simulink model "pacemaker"  (R2020a)
settings: Solver=FixedStepAuto  StartTime=0.0  StopTime=10.0  FixedStep=1e-3  RelTol=1e-3  EnableMultiTasking=on
undefined symbols (not defined in the file): A0, A1, D0, D1, D10, D11, D12, D13, D2, D3, D4, D5, D6, D7, D8, D9, PTA0, PTA1, PTA2, PTB2, PTB23, PTB3, PTB9, PTC16, PTC17, PTC2, PTC3, PTC4, PTD0, PTD1, PTD2, PTD3
libraries: frdmk64flib x22, etargetslib x8
settings Model: ExtModeTrigDuration=5  Creator=V  LastModifiedBy=V
settings OptimizationCC: EnhancedBackFolding=on  PassReuseOutputArgsAs=Individual arguments  ZeroExternalMemoryAtStartup=off  ZeroInternalMemoryAtStartup=off  MaxStackSize=64  OptimizeBlockOrder=speed  DifferentSizesBufferReuse=on  OptimizationCustomize=off  EfficientTunableParamExpr=on
settings DebuggingCC: ParameterTunabilityLossMsg=error
settings HardwareCC: ProdBitPerPointer=32  ProdBitPerSizeT=32  ProdBitPerPtrDiffT=32  ProdLargestAtomicInteger=Long  ProdLargestAtomicFloat=Double  ProdWordSize=32  ProdHWDeviceType=ARM Compatible->ARM Cortex
settings SFSimCC: MATLABDynamicMemAlloc=off
settings RTWCC: SystemTargetFile=ert.tlc  HardwareBoard=NXP FRDM-K64F  TemplateMakefile=ert_default_tmf  Toolchain=GNU Tools for ARM Embedded Processors
settings CodeAppCC: ForceParamTrailComments=on  IgnoreCustomStorageClasses=off  OperatorAnnotations=on  SimulinkDataObjDesc=on  SFDataObjDesc=on  InsertBlockDesc=on

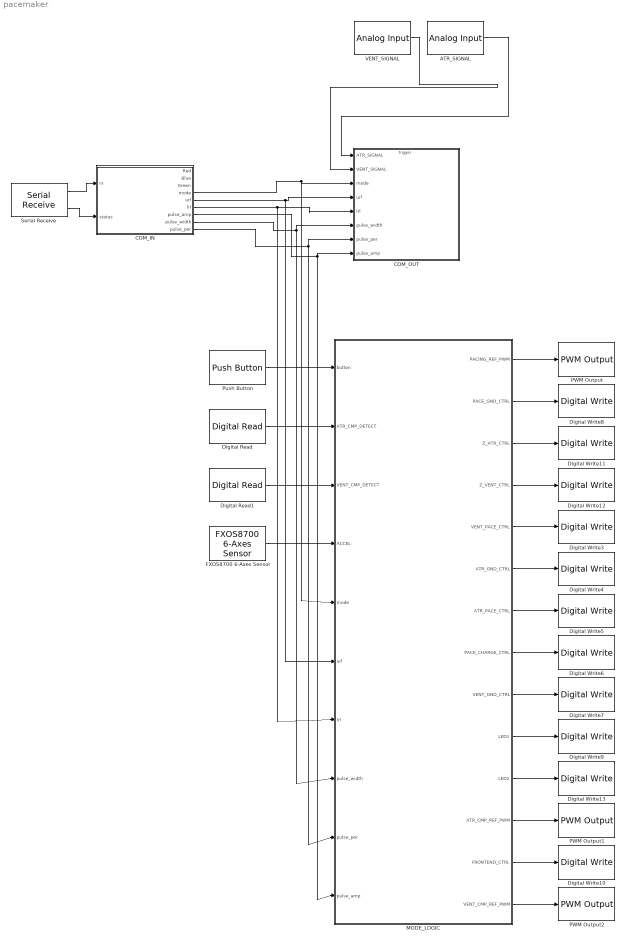
== system pacemaker ==
  ATR_SIGNAL : frdmk64flib/Analog Input  Whichpin=PTB2 (A0)  SampleTime=-1
  COM_IN : Stateflow chart  TreatAsAtomicUnit=on
      settings: PortSchema="{\"entries\":[{\"content\":{\"sides\":[{\"content\":{\"connectorIds\":[\"In2\",\"In1\"]},\"type\":\"ConnectorPlacement.EquallySpacedRectSide\",\"uuid\":\"8daf93b5-21b0-4142-b4ab-857b16f8f8fd\"},{\"content\":{\"connectorIds\":[\"Out1\",\"Out2\",\"Out3\",\"Out4\",\"Out5\",\"Out6\",\"Out7\",\"Out8\",\"Out9\"],\"side\":\"RIGHT\"},\"type\":\"ConnectorPlacement.EquallySpacedRectSide\",\"uuid\":\"6413e42a-ae9b-49fc-8e61-a3b5f4c35bed\"},{\"content\":{\"connectorIds\":[],\"side\":\"TOP\"},\"type\":\"ConnectorPlacement.EquallySpacedRectSide\",\"uuid\":\"39f92d96-10a7-4496-b9ea-08b56c7f9280\"}]},\"type\":\"ConnectorPlacement.EquallySpacedConnector\",\"uuid\":\"717f6531-5e3e-445a-90fb-8047e6ab3765\"}],\"packageUris\":[\"http://schema.mathworks.com/mf0/Connector/19700101\"],\"version\":\"1.0\"}"
  COM_OUT : Subsystem
  Digital Read : frdmk64flib/Digital Read  Whichpin=PTC16 (D0)  SampleTime=-1
  Digital Read1 : frdmk64flib/Digital Read  Whichpin=PTC17 (D1)  SampleTime=-1
  Digital Write10 : frdmk64flib/Digital Write  Whichpin=PTD1 (D13)
  Digital Write11 : frdmk64flib/Digital Write  Whichpin=PTB23 (D4)
  Digital Write12 : frdmk64flib/Digital Write  Whichpin=PTC3 (D7)
  Digital Write13 : frdmk64flib/Digital Write  Whichpin=GREEN_LED
  Digital Write3 : frdmk64flib/Digital Write  Whichpin=PTC4 (D9)
  Digital Write4 : frdmk64flib/Digital Write  Whichpin=PTD2 (D11)
  Digital Write5 : frdmk64flib/Digital Write  Whichpin=PTA0 (D8)
  Digital Write6 : frdmk64flib/Digital Write  Whichpin=PTB9 (D2)
  Digital Write7 : frdmk64flib/Digital Write  Whichpin=PTD3 (D12)
  Digital Write8 : frdmk64flib/Digital Write  Whichpin=PTD0 (D10)
  Digital Write9 : frdmk64flib/Digital Write  Whichpin=RED_LED
  FXOS8700 6-Axes Sensor : frdmk64flib/FXOS8700 6-Axes Sensor  Activesensor=Accelerometer only  ODR=800Hz  HybridODR=400Hz  Accelfullrange=-4g to +4g  SampleTime=-1
  MODE_LOGIC : Stateflow chart  TreatAsAtomicUnit=on
      settings: PortSchema="{\"entries\":[{\"content\":{\"sides\":[{\"content\":{\"connectorIds\":[\"In1\",\"In2\",\"In3\",\"In4\",\"In10\",\"In6\",\"In5\",\"In8\",\"In7\",\"In9\"]},\"type\":\"ConnectorPlacement.EquallySpacedRectSide\",\"uuid\":\"04414c83-1a99-45b4-b483-67b067b91455\"},{\"content\":{\"connectorIds\":[\"Out1\",\"Out2\",\"Out3\",\"Out4\",\"Out5\",\"Out6\",\"Out7\",\"Out8\",\"Out9\",\"Out10\",\"Out11\",\"Out12\",\"Out13\",\"Out14\"],\"side\":\"RIGHT\"},\"type\":\"ConnectorPlacement.EquallySpacedRectSide\",\"uuid\":\"10735fb8-9010-49d7-9ae9-fd379b89587a\"},{\"content\":{\"connectorIds\":[],\"side\":\"TOP\"},\"type\":\"ConnectorPlacement.EquallySpacedRectSide\",\"uuid\":\"3c1ca38a-0b4c-49c9-8ccc-830417faf6d4\"}]},\"type\":\"ConnectorPlacement.EquallySpacedConnector\",\"uuid\":\"9d19b875-14af-4a64-aa13-2b0c973f73dc\"}],\"packageUris\":[\"http://schema.mathworks.com/mf0/Connector/19700101\"],\"version\":\"1.0\"}"
  PWM Output : frdmk64flib/PWM Output  Whichpin=PTA2 (D5)  InitialFrequency=2000  InitialDutyCycle=70
  PWM Output1 : frdmk64flib/PWM Output  Whichpin=PTC2 (D6)  InitialFrequency=2000  InitialDutyCycle=50
  PWM Output2 : frdmk64flib/PWM Output  Whichpin=PTA1 (D3)  InitialFrequency=2000  InitialDutyCycle=50
  Push Button : frdmk64flib/Push Button  Whichswitch=SW2  SampleTime1=-1
  Serial Receive : frdmk64flib/Serial Receive  SCIModule=0  Baudrate=uint32(9600)  Parity=None  StopBits=1  HardwareFlowControl=None  ByteOrder=LittleEndian  DataType=uint8  DataLength=44  BlockingMode=off  OutputStatus=on  SampleTime=0.1
  VENT_SIGNAL : frdmk64flib/Analog Input  Whichpin=PTB3 (A1)  SampleTime=-1
  wires:
  Serial Receive/2 -> COM_IN/1(status)
  Serial Receive/1 -> COM_IN/2(rx)
  VENT_SIGNAL/1 -> COM_OUT/2(VENT_SIGNAL)
  ATR_SIGNAL/1 -> COM_OUT/1(ATR_SIGNAL)
  COM_IN/4(mode) -> MODE_LOGIC/10(mode), COM_OUT/3(mode)
  COM_IN/5(url) -> MODE_LOGIC/6(url), COM_OUT/4(url)
  COM_IN/6(lrl) -> MODE_LOGIC/5(lrl), COM_OUT/5(lrl)
  COM_IN/8(pulse_width) -> MODE_LOGIC/8(pulse_width), COM_OUT/6(pulse_width)
  COM_IN/7(pulse_amp) -> MODE_LOGIC/9(pulse_amp), COM_OUT/8(pulse_amp)
  COM_IN/9(pulse_per) -> MODE_LOGIC/7(pulse_per), COM_OUT/7(pulse_per)
  MODE_LOGIC/8(PACE_CHARGE_CTRL) -> Digital Write6/1
  MODE_LOGIC/10(LED1) -> Digital Write9/1
  MODE_LOGIC/6(ATR_GND_CTRL) -> Digital Write4/1
  MODE_LOGIC/13(FRONTEND_CTRL) -> Digital Write10/1
  MODE_LOGIC/2(PACE_GND_CTRL) -> Digital Write8/1
  MODE_LOGIC/9(VENT_GND_CTRL) -> Digital Write7/1
  MODE_LOGIC/14(VENT_CMP_REF_PWM) -> PWM Output2/1
  MODE_LOGIC/7(ATR_PACE_CTRL) -> Digital Write5/1
  MODE_LOGIC/1(PACING_REF_PWM) -> PWM Output/1
  MODE_LOGIC/11(LED2) -> Digital Write13/1
  MODE_LOGIC/12(ATR_CMP_REF_PWM) -> PWM Output1/1
  MODE_LOGIC/3(Z_ATR_CTRL) -> Digital Write11/1
  MODE_LOGIC/4(Z_VENT_CTRL) -> Digital Write12/1
  MODE_LOGIC/5(VENT_PACE_CTRL) -> Digital Write3/1
  Push Button/1 -> MODE_LOGIC/1(button)
  Digital Read/1 -> MODE_LOGIC/2(ATR_CMP_DETECT)
  Digital Read1/1 -> MODE_LOGIC/3(VENT_CMP_DETECT)
  FXOS8700 6-Axes Sensor/1 -> MODE_LOGIC/4(ACCEL)

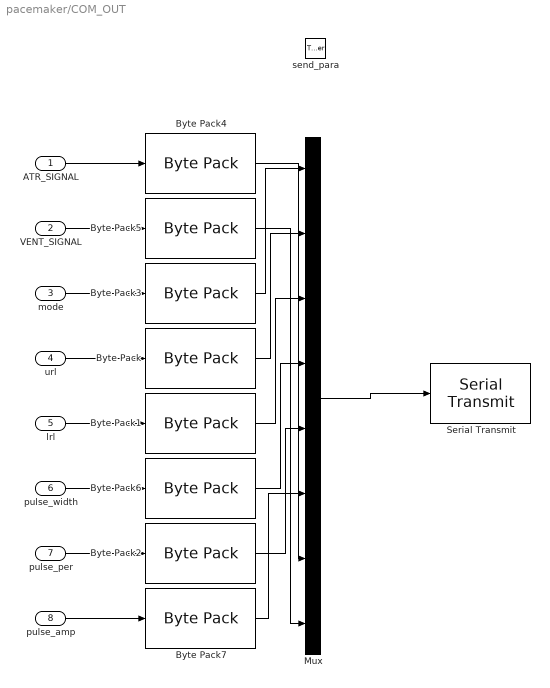
== system pacemaker/COM_OUT ==
  ATR_SIGNAL : Inport  OutDataTypeStr=double
  VENT_SIGNAL : Inport  Port=2  OutDataTypeStr=double
  mode : Inport  Port=3  OutDataTypeStr=uint16
  url : Inport  Port=4  OutDataTypeStr=double
  lrl : Inport  Port=5  OutDataTypeStr=double
  pulse_width : Inport  Port=6  OutDataTypeStr=double
  pulse_per : Inport  Port=7  OutDataTypeStr=double
  pulse_amp : Inport  Port=8  OutDataTypeStr=double
  send_para : TriggerPort  TriggerType=function-call  IsSimulinkFunction=on  FunctionName=send_para  VariantControl=Variant
  Byte Pack{,1..2,4..7} (7 alike) : etargetslib/Byte Pack  datatypes={'double'}  byteAlign=1
  Byte Pack3 : etargetslib/Byte Pack  datatypes={'uint16'}  byteAlign=1
  Mux : Mux  Inputs=8
  Serial Transmit : frdmk64flib/Serial Transmit  SCIModule=0  Baudrate=uint32(9600)  Parity=None  StopBits=1  HardwareFlowControl=None  ByteOrder=LittleEndian  BlockingMode=on  OutputStatus=off
  wires:
  Mux/1 -> Serial Transmit/1
  ATR_SIGNAL/1 -> Byte Pack4/1
  VENT_SIGNAL/1 -> Byte Pack5/1
  Byte Pack7/1 -> Mux/6
  Byte Pack6/1 -> Mux/4
  url/1 -> Byte Pack/1
  lrl/1 -> Byte Pack1/1
  Byte Pack/1 -> Mux/2
  Byte Pack1/1 -> Mux/3
  mode/1 -> Byte Pack3/1
  Byte Pack2/1 -> Mux/5
  pulse_amp/1 -> Byte Pack7/1
  pulse_per/1 -> Byte Pack2/1
  pulse_width/1 -> Byte Pack6/1
  Byte Pack3/1 -> Mux/1
  Byte Pack5/1 -> Mux/8
  Byte Pack4/1 -> Mux/7

== stateflow chart pacemaker/MODE_LOGIC ==
  state Capacitor_Charge_ [commented out]
    entry:
    ATR_PACE_CTRL = false;
    VENT_PACE_CTRL = false;
    PACING_REF_PWM =70;
    PACE_CHARGE_CTRL = true;
    %delay
    %pulse_width = 0.4;
    pulse_amp = 0.5;
    %fixed_delay = 150;
    %vref_per = 320;
    %aref_per = 250;
    %LRL = 60;
    %URL = 120;
    PACE_GND_CTRL = true;
    VENT_PACE_CTRL = false;
    Z_ATR_CTRL = false;
    Z_VENT_CTRL = false;
    if(mode ==0)
    ATR_PACE_CTRL = false;
    ATR_GND_CTRL = true;
    VENT_GND_CTRL = false;
    elseif(mode ==1)
    VENT_PACE_CTRL = false;
    VENT_GND_CTRL = true;
    ATR_GND_CTRL = false;
    end
    ATR_CMP_REF_PWM = 99;
    VENT_CMP_REF_PWM = 99;
    FRONTEND_CTRL = true;
    acceleration = sqrt(ACCEL(1)^2+ACCEL(2)^2);
    if(acceleration>0.75)
    LED1 = true;
    LED2=false;
    else
    LED1= false;
    LED2 = true;
    end
  state AOO [commented out]
    entry:
    PACE_CHARGE_CTRL= false;
    PACING_REF_PWM =0;
    if(mode ==1)
    ATR_PACE_CTRL= true;
    ATR_GND_CTRL = false;
    VENT_GND_CTRL = false;
    mode = 0;
    elseif(mode ==0)
    VENT_PACE_CTRL = true;
    VENT_GND_CTRL = false;
    ATR_GND_CTRL = false;
    mode = 1;
    end
    Z_ATR_CTRL = false;
    Z_VENT_CTRL = false;
    %delay
  state AOO_AOOR
    entry:
    PACE_CHARGE_CTRL= false;
    ATR_PACE_CTRL= true;
    ATR_GND_CTRL = false;
    Z_ATR_CTRL = false;
    Z_VENT_CTRL = false;
    %delay
  state Capacitor_Charge_1
    entry:
    ATR_PACE_CTRL = false;
    VENT_PACE_CTRL = false;
    PACING_REF_PWM =int32((pulse_amp/5)*100);
    PACE_CHARGE_CTRL = true;
    %Below are parameters I am asking the TA about
    %fixed_delay = 150;
    %vref_per = 320;
    %aref_per = 250;
    %Programmable Parameters are:
    %lrl
    %url
    %pulse_width
    %pulse_per
    %pulse_amp
    %right now these are all local data, but should be changed to input data
    LRL = 1000*60/lrl;
    URL = 1000*60/url;
    MODE = mode;
    PACE_GND_CTRL = true;
    VENT_PACE_CTRL = false;
    Z_ATR_CTRL = false;
    Z_VENT_CTRL = false;
    ATR_PACE_CTRL = false;
    if(MODE == 2 | MODE==4| (MODE==5|MODE==10)&dual_mode==1|MODE==7|MODE==9)
    ATR_GND_CTRL = false;
    VENT_GND_CTRL = true;
    elseif(MODE ==1 | MODE ==3|MODE==5|MODE==10|MODE==6|MODE==8)
    ATR_GND_CTRL = true;
    VENT_GND_CTRL = false;
    end
    if(button == true &MODE<10)
    MODE = MODE +1;
    elseif(button == true & MODE ==10)
    MODE = 1;
    end
    LED2 = true;
    LED1 = false;
    ATR_CMP_REF_PWM = 70;
    VENT_CMP_REF_PWM = 70;
    FRONTEND_CTRL = true;
    acceleration = sqrt(ACCEL(1)^2+ACCEL(2)^2);
    if(mode>5)
    if(acceleration<0.75)
    rate=LRL-(LRL-URL)*(acceleration/0.75);
    else
    rate = URL;
    end
    end
  state VOO_VOOR
    entry:
    PACE_CHARGE_CTRL= false;
    VENT_PACE_CTRL = true;
    VENT_GND_CTRL = false;
    Z_ATR_CTRL = false;
    Z_VENT_CTRL = false;
    %delay
  state DOO_DOOR
    entry:
    PACE_CHARGE_CTRL= false;
    PACING_REF_PWM =0;
    if(dual_mode ==1)
    ATR_PACE_CTRL= true;
    ATR_GND_CTRL = false;
    VENT_GND_CTRL = false;
    dual_mode = 0;
    elseif(dual_mode ==0)
    VENT_PACE_CTRL = true;
    VENT_GND_CTRL = false;
    ATR_GND_CTRL = false;
    dual_mode = 1;
    end
    Z_ATR_CTRL = false;
    Z_VENT_CTRL = false;
    %delay
  state AAI_AAIR_VVI_VVIR
    state Wait
      entry:
      LED2=false;
    state AAI_AAIR
      entry:
      PACE_CHARGE_CTRL= false;
      ATR_PACE_CTRL= true;
      ATR_GND_CTRL = false;
      Z_ATR_CTRL = false;
      Z_VENT_CTRL = false;
      %delay
      LED1 = true;
      LED2 = false;
    state VVI_VVIR
      entry:
      PACE_CHARGE_CTRL= false;
      VENT_PACE_CTRL = true;
      VENT_GND_CTRL = false;
      Z_ATR_CTRL = false;
      Z_VENT_CTRL = false
      %delay
      LED1 = true;
      LED2 = false;
    Wait -> Wait [order 2] : [(ATR_CMP_DETECT==true&(mode==3|mode==8))|(VENT_CMP_DETECT==true&(mode==4|mode==9))]
    Wait -> AAI_AAIR [order 1] : [(mode==3 &after(pulse_per,msec)&ATR_CMP_DETECT==false)|(mode==8 &after(rate,msec)&ATR_CMP_DETECT==false)]
    Wait -> VVI_VVIR [order 3] : [(mode==4&after(pulse_per,msec)&VENT_CMP_DETECT==false)|(mode==9&after(rate,msec)&VENT_CMP_DETECT==false)]
  Capacitor_Charge_1 -> Wait [order 3] : [MODE==3 |MODE ==4|MODE==8|MODE==9]%signal detected
  (default) -> Capacitor_Charge_ [commented out]
  AOO -> Capacitor_Charge_ [commented out] : [after(10,msec)]
  Capacitor_Charge_ -> AOO [commented out] : [after(1000,msec)]
  AOO_AOOR -> Capacitor_Charge_1 : [(MODE == 1|MODE==6)&after(pulse_width,msec)]
  Capacitor_Charge_1 -> AOO_AOOR [order 1] : [MODE == 1&after(pulse_per,msec)|MODE==6&after(rate,msec)]
  (default) -> Capacitor_Charge_1
  Capacitor_Charge_1 -> VOO_VOOR [order 2] : [MODE == 2&after(pulse_per,msec)|MODE==7&after(rate,msec)]
  Capacitor_Charge_1 -> DOO_DOOR [order 4] : [(MODE==5&after(pulse_per/2,msec))|(MODE==10&after(rate/2,msec))]
  VOO_VOOR -> Capacitor_Charge_1 : [(MODE == 2|MODE==7)&after(pulse_width,msec)]
  DOO_DOOR -> Capacitor_Charge_1 : [(MODE==5|MODE==10)&after(pulse_width,msec)]
  VVI_VVIR -> Capacitor_Charge_1 : [after(pulse_width,msec)]
  AAI_AAIR -> Capacitor_Charge_1 : [after(pulse_width,msec)]
  data: PACING_REF_PWM output int32; PACE_GND_CTRL output boolean; Z_ATR_CTRL output boolean; Z_VENT_CTRL output boolean; VENT_PACE_CTRL output boolean; ATR_GND_CTRL output boolean; ATR_PACE_CTRL output boolean; PACE_CHARGE_CTRL output boolean; VENT_GND_CTRL output boolean; button input boolean; LED1 output boolean; LED2 output boolean; ATR_CMP_DETECT input boolean; ATR_CMP_REF_PWM output double; FRONTEND_CTRL output boolean; PULSE local boolean; counter local double =0; x local; VENT_CMP_REF_PWM output int32; VENT_CMP_DETECT input boolean; ACCEL input double size=[1 3]; acceleration local double =0; dual_mode local double =0; rate local double =1000; LRL local double; URL local double; lrl input double =60; url input double =120; pulse_per input double =1000; pulse_width input double =10; pulse_amp input double =5; mode input uint16 =1; MODE local uint16

== stateflow chart pacemaker/COM_IN ==
  state Action
    entry:
    pulse_amp = typecast(rx(3:10),'double')
    pulse_width = typecast(rx(11:18),'double')
    pulse_per = typecast(rx(19:26),'double')
    lrl = typecast(rx(27:34),'double')
    url = typecast(rx(35:42),'double')
    mode = typecast(rx(43:44),'uint16')
  state Init
    entry:
    mode = 1;
    url=120;
    lrl=60;
    pulse_amp = 5;
    pulse_width = 10;
    pulse_per = 1000;
    Red = 1;
    Blue = 0;
    Green = 0;
  state Stand
  state Echo
    entry:
    send_para();
    Blue = 1;
  (default) -> Init
  Action -> Stand
  (junction 7) -> Action [order 1] : [rx(2) == hex2dec('55')]
  (junction 6) -> Stand [order 2]
  Init -> Stand
  Stand -> (junction 6) : [status == 0]
  (junction 6) -> (junction 7) [order 1] : [rx(1) == hex2dec('16')]
  (junction 7) -> Echo [order 2] : [rx(2) == hex2dec('22')]
  Echo -> Stand
  data: status input uint8; rx input uint8; Red output; Blue output; Green output; mode output uint16; url output double; lrl output double; pulse_amp output double; pulse_width output double; pulse_per output double
